simulink model "Segundo"  (R2017b)
settings: Solver=VariableStepAuto  StartTime=0.0  StopTime=0.03  RelTol=1e-3
values from neighbouring files (symbols this model uses):
  kd = eval(S.kd)    [Cuarto_P_I_D.m]    (also in Quinto_P_I_D.m; Segundoo.m; SeptimoBPIDD2.m; SeptimoPIDD2.m)
  ki = eval(S.ki)    [Cuarto_P_I_D.m]    (also in Quinto_P_I_D.m; Segundoo.m; SeptimoBPIDD2.m; SeptimoPIDD2.m)
  kp = eval(S.kp)    [Cuarto_P_I_D.m]    (also in Quinto_P_I_D.m; Segundoo.m; SeptimoBPIDD2.m; SeptimoPIDD2.m)
settings Model: Creator=Cx001la  LastModifiedBy=Cx001la

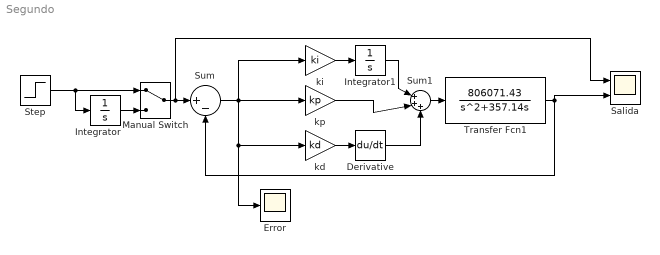
== system Segundo ==
  Derivative : Derivative
  Error : Scope
  Integrator : Integrator
  Integrator1 : Integrator
  Manual Switch : ManualSwitch
  Salida : Scope  NumInputPorts=2
  Step : Step  Time=0  SampleTime=0
  Sum : Sum  Inputs=|+-
  Sum1 : Sum  Inputs=|+++
  Transfer Fcn1 : TransferFcn  Numerator=[806071.43]  Denominator=[1 357.14 0]
  kd : Gain  Gain=kd
  ki : Gain  Gain=ki
  kp : Gain  Gain=kp
  wires:
  Transfer Fcn1/1 -> Sum/2, Salida/2
  Step/1 -> Integrator/1, Manual Switch/1
  Manual Switch/1 -> Salida/1, Sum/1
  Integrator/1 -> Manual Switch/2
  Sum/1 -> kd/1, Error/1, kp/1, ki/1
  ki/1 -> Integrator1/1
  kd/1 -> Derivative/1
  Sum1/1 -> Transfer Fcn1/1
  Integrator1/1 -> Sum1/1
  kp/1 -> Sum1/2
  Derivative/1 -> Sum1/3
